simulink model "MorseCode"  (R2013b)
settings: Solver=FixedStepDiscrete  SolverMode=SingleTasking  StartTime=0.0  StopTime=10.0  FixedStep=0.25  RelTol=1e-3
libraries: arduinolib x3
settings Model: ExtModeTrigDuration=2  Creator=ian.alferez  LastModifiedBy=ian.alferez
settings OptimizationCC: OptimizeModelRefInitCode=on  LifeSpan=1
settings DebuggingCC: SolverPrmCheckMsg=none
settings HardwareCC: ProdBitPerInt=16  ProdBitPerPointer=8  ProdIntDivRoundTo=Zero  ProdEndianess=LittleEndian  ProdWordSize=8  ProdHWDeviceType=Atmel->AVR
settings RTWCC: SystemTargetFile=realtime.tlc  GenerateMakefile=off  TemplateMakefile=realtime.tmf  Description=Run on Target Hardware  RTWVerbose=off  ProcessScript=realtime_make_rtw_hook
settings STFCustomTargetCC: TargetLibSuffix=.a  GenerateSampleERTMain=on  ERTCustomFileBanners=on  SupportNonInlinedSFcns=off  SupportVariableSizeSignals=on  MATLABClassNameForMDSCustomization=Simulink.SoftwareTarget.ERTCustomization  GRTInterface=off  SystemTargetFile=realtime.tlc
settings ERTTargetCC: CodeReplacementLibrary=ANSI_C  GenerateSampleERTMain=on  ParMdlRefBuildCompliant=off  CompOptLevelCompliant=off  ConcurrentExecutionCompliant=off  CombineOutputUpdateFcns=off  ERTFirstTimeCompliant=off  SupportContinuousTime=on  SupportVariableSizeSignals=on  ModelStepFunctionPrototypeControlCompliant=off  CPPClassGenCompliant=off  ExtModeTransport=3  ExtModeMexFile=ext_serial_win32_comm  ExtModeMexArgs=0 1 9600  InlinedParameterPlacement=NonHierarchical  ERTSrcFileBannerTemplate=realtime_code_template.cgt  ERTHdrFileBannerTemplate=realtime_code_template.cgt  ERTDataSrcFileTemplate=realtime_code_template.cgt  ERTDataHdrFileTemplate=realtime_code_template.cgt  ERTCustomFileTemplate=realtime_file_process.tlc

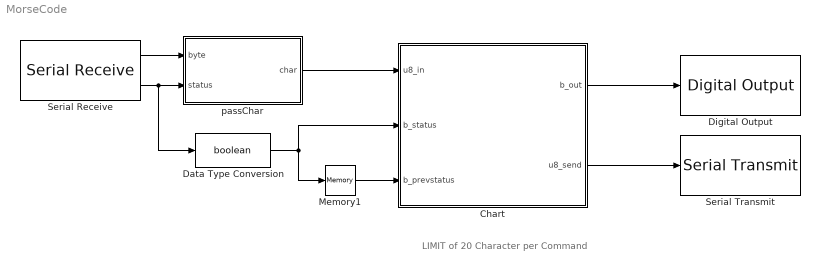
== system MorseCode ==
  note: LIMIT of 20 Character per Command
  Chart : Stateflow chart  TreatAsAtomicUnit=on
  Data Type Conversion : DataTypeConversion  OutDataTypeStr=boolean
  Digital Output : arduinolib/Digital Output  pinNumber=13
  Memory1 : Memory
  Serial Receive : arduinolib/Serial Receive  portNumber=0  showOutStatus=on  sampleTime=0.5
  Serial Transmit : arduinolib/Serial Transmit  portNumber=0
  passChar : MATLAB Function  TreatAsAtomicUnit=on
  wires:
  Serial Receive/2 -> Data Type Conversion/1, passChar/2(status)
  Serial Receive/1 -> passChar/1(byte)
  passChar/1(char) -> Chart/1(u8_in)
  Chart/1(b_out) -> Digital Output/1
  Data Type Conversion/1 -> Memory1/1, Chart/2(b_status)
  Memory1/1 -> Chart/3(b_prevstatus)
  Chart/2(u8_send) -> Serial Transmit/1

== matlab function MorseCode/passChar ==
  data: byte input; char output; status input
function char = passChar(byte,status)
%#codegen
persistent last

if isempty(last)
    last = uint8(0);
end

if (byte>=0 && status == 1)
    last = byte;
else
    byte = last;
end

char = uint8(byte);

== stateflow chart MorseCode/Chart ==
  state SOURCE_MAIN [parallel]
    settings: executionOrder=1
    state RUN
      state STARTUP
      state DONE
        entry:
        b_gotomain = TRUE;
      (default) -> STARTUP : {
          | u8_counter = 0;
          | u8_character[0] = 0;
          | u8_character[1] = 0;
          | u8_character[2] = 0;
          | u8_character[3] = 0;
          | u8_character[4] = 0;
          | u8_character[5] = 0;
          | u8_character[6] = 0;
          | u8_character[7] = 0;
          | u8_character[8] = 0;
          | u8_character[9] = 0;
          | u8_character[10] = 0;
          | u8_character[11] = 0;
          | u8_character[12] = 0;
          | u8_character[13] = 0;
          | u8_character[14] = 0;
          | u8_character[15] = 0;
          | u8_character[16] = 0;
          | u8_character[17] = 0;
          | u8_character[18] = 0;
          | u8_character[19] = 0;
          | }
      STARTUP -> (junction 10)
      (junction 10) -> (junction 3) [order 1] : [b_status == TRUE &&...
          | b_prevstatus == FALSE]
      (junction 10) -> (junction 14) [order 2]
      (junction 3) -> (junction 6) : {
          | u8_character[u8_counter] = u8_in;
          | u8_counter += 1;
          | }
      (junction 6) -> (junction 14) [order 2]
      (junction 6) -> DONE [order 1] : [u8_in == 13]
      (junction 14) -> (junction 39)
    state MAIN
      state Process
        entry:
        b_out = 0;
        u8_count = 0;
        state PULSE
          state IDLE
            b_end = FALSE;
          state SHORT_1
            entry:
            u8_count = 0;
            state OFF
              entry:
              b_out = 0;
            state ON
              entry:
              b_out =1;
              u8_count += 1;
            (default) -> SOURCE_MAIN.MAIN.Process.PULSE.SHORT_1.OFF
            SOURCE_MAIN.MAIN.Process.PULSE.SHORT_1.OFF -> SOURCE_MAIN.MAIN.Process.PULSE.SHORT_1.ON : after(0.25, sec)
            SOURCE_MAIN.MAIN.Process.PULSE.SHORT_1.ON -> SOURCE_MAIN.MAIN.Process.PULSE.SHORT_1.OFF : after(0.25, sec)
          state LONG_1
            entry:
            u8_count = 0;
            state OFF
              entry:
              b_out = 0;
            state ON
              entry:
              b_out =1;
              u8_count += 1;
            (default) -> SOURCE_MAIN.MAIN.Process.PULSE.LONG_1.OFF
            SOURCE_MAIN.MAIN.Process.PULSE.LONG_1.OFF -> SOURCE_MAIN.MAIN.Process.PULSE.LONG_1.ON : after(0.25, sec)
            SOURCE_MAIN.MAIN.Process.PULSE.LONG_1.ON -> SOURCE_MAIN.MAIN.Process.PULSE.LONG_1.OFF : after(1, sec)
          state SHORT_2
            entry:
            u8_count = 0;
            state OFF
              entry:
              b_out = 0;
            state ON
              entry:
              b_out =1;
              u8_count += 1;
            (default) -> SOURCE_MAIN.MAIN.Process.PULSE.SHORT_2.OFF
            SOURCE_MAIN.MAIN.Process.PULSE.SHORT_2.OFF -> SOURCE_MAIN.MAIN.Process.PULSE.SHORT_2.ON : after(0.25, sec)
            SOURCE_MAIN.MAIN.Process.PULSE.SHORT_2.ON -> SOURCE_MAIN.MAIN.Process.PULSE.SHORT_2.OFF : after(0.25, sec)
          state LONG_2
            entry:
            u8_count = 0;
            state OFF
              entry:
              b_out = 0;
            state ON
              entry:
              b_out =1;
              u8_count += 1;
            (default) -> SOURCE_MAIN.MAIN.Process.PULSE.LONG_2.OFF
            SOURCE_MAIN.MAIN.Process.PULSE.LONG_2.OFF -> SOURCE_MAIN.MAIN.Process.PULSE.LONG_2.ON : after(0.25, sec)
            SOURCE_MAIN.MAIN.Process.PULSE.LONG_2.ON -> SOURCE_MAIN.MAIN.Process.PULSE.LONG_2.OFF : after(1, sec)
          state SHORT_3
            entry:
            u8_count = 0;
            state OFF
              entry:
              b_out = 0;
            state ON
              entry:
              b_out =1;
              u8_count += 1;
            (default) -> SOURCE_MAIN.MAIN.Process.PULSE.SHORT_3.OFF
            SOURCE_MAIN.MAIN.Process.PULSE.SHORT_3.OFF -> SOURCE_MAIN.MAIN.Process.PULSE.SHORT_3.ON : after(0.25, sec)
            SOURCE_MAIN.MAIN.Process.PULSE.SHORT_3.ON -> SOURCE_MAIN.MAIN.Process.PULSE.SHORT_3.OFF : after(0.25, sec)
          state LONG_3
            entry:
            u8_count = 0;
            state OFF
              entry:
              b_out = 0;
            state ON
              entry:
              b_out =1;
              u8_count += 1;
            (default) -> SOURCE_MAIN.MAIN.Process.PULSE.LONG_3.OFF
            SOURCE_MAIN.MAIN.Process.PULSE.LONG_3.OFF -> SOURCE_MAIN.MAIN.Process.PULSE.LONG_3.ON : after(0.25, sec)
            SOURCE_MAIN.MAIN.Process.PULSE.LONG_3.ON -> SOURCE_MAIN.MAIN.Process.PULSE.LONG_3.OFF : after(1, sec)
          state SHORT_4
            entry:
            u8_count = 0;
            state OFF
              entry:
              b_out = 0;
            state ON
              entry:
              b_out =1;
              u8_count += 1;
            (default) -> SOURCE_MAIN.MAIN.Process.PULSE.SHORT_4.OFF
            SOURCE_MAIN.MAIN.Process.PULSE.SHORT_4.OFF -> SOURCE_MAIN.MAIN.Process.PULSE.SHORT_4.ON : after(0.25, sec)
            SOURCE_MAIN.MAIN.Process.PULSE.SHORT_4.ON -> SOURCE_MAIN.MAIN.Process.PULSE.SHORT_4.OFF : after(0.25, sec)
          state LONG_4
            entry:
            u8_count = 0;
            state OFF
              entry:
              b_out = 0;
            state ON
              entry:
              b_out =1;
              u8_count += 1;
            (default) -> SOURCE_MAIN.MAIN.Process.PULSE.LONG_4.OFF
            SOURCE_MAIN.MAIN.Process.PULSE.LONG_4.OFF -> SOURCE_MAIN.MAIN.Process.PULSE.LONG_4.ON : after(0.25, sec)
            SOURCE_MAIN.MAIN.Process.PULSE.LONG_4.ON -> SOURCE_MAIN.MAIN.Process.PULSE.LONG_4.OFF : after(1, sec)
          state END
            entry:
            b_end = TRUE;
            u8_count1 += 1;
          (default) -> SOURCE_MAIN.MAIN.Process.PULSE.IDLE
          SOURCE_MAIN.MAIN.Process.PULSE.IDLE -> (junction 48)
          (junction 48) -> (junction 49) [order 1] : [(u8_long1_count > 0) && (u8_short1_count == 0)]
          (junction 48) -> SHORT_1 [order 2]
          (junction 49) -> LONG_1
          SHORT_1 -> (junction 50) : [(u8_count >= u8_short1_count) && (b_out == 0)]
          LONG_1 -> (junction 51) : [(u8_count >= u8_long1_count) && (b_out == 0)]
          (junction 51) -> (junction 50)
          (junction 50) -> (junction 52)
          (junction 52) -> (junction 53) [order 1] : [(u8_long2_count > 0) && (u8_short2_count == 0)]
          (junction 52) -> SHORT_2 [order 2]
          (junction 53) -> LONG_2
          SHORT_2 -> (junction 54) : [(u8_count >= u8_short2_count) && (b_out == 0)]
          LONG_2 -> (junction 55) : [(u8_count >= u8_long2_count) && (b_out == 0)]
          (junction 55) -> (junction 54)
          (junction 54) -> (junction 56)
          (junction 56) -> (junction 57) [order 1] : [(u8_long3_count > 0) && (u8_short3_count == 0)]
          (junction 56) -> SHORT_3 [order 2]
          (junction 57) -> LONG_3
          SHORT_3 -> (junction 58) : [(u8_count >= u8_short3_count) && (b_out == 0)]
          LONG_3 -> (junction 59) : [(u8_count >= u8_long3_count) && (b_out == 0)]
          (junction 59) -> (junction 58)
          (junction 58) -> (junction 60)
          (junction 60) -> (junction 61) [order 1] : [(u8_long4_count > 0) && (u8_short4_count == 0)]
          (junction 60) -> SHORT_4 [order 2]
          (junction 61) -> LONG_4
          SHORT_4 -> (junction 62) : [(u8_count >= u8_short4_count) && (b_out == 0)]
          LONG_4 -> (junction 63) : [(u8_count >= u8_long4_count) && (b_out == 0)]
          (junction 63) -> (junction 62)
          (junction 62) -> END
        (default) -> PULSE : {
            | [u8_long1_count,u8_short1_count,...
            | u8_long2_count,u8_short2_count,...
            | u8_long3_count,u8_short3_count,...
            | u8_long4_count,u8_short4_count] = convert(u8_character[u8_count1]);
            | }
      state IDLE
        entry:
        b_end = FALSE;
      (default) -> SOURCE_MAIN.MAIN.IDLE : {
          | b_end = FALSE;
          | u8_count1 = 0;
          | }
      SOURCE_MAIN.MAIN.IDLE -> Process : [b_end == FALSE]
      Process -> SOURCE_MAIN.MAIN.IDLE : [b_end == TRUE]
    (default) -> RUN : {b_gotomain = FALSE;}
    RUN -> MAIN : [b_gotomain == TRUE]
    MAIN -> (junction 179) : [b_end == TRUE && ...
        | u8_count1 >= u8_counter]
    (junction 179) -> (junction 180) : {
        | b_gotomain = FALSE;
        | }
    (junction 180) -> RUN
  state SOURCE_TRANSMIT [parallel]
    settings: executionOrder=2
    state INIT
    state NEWLINE
      entry:
      u8_send = 10;
    state CHAR
      entry:
      u8_send = u8_in;
    state ENTER
      entry:
      u8_send = 13;
    state NULL
      entry:
      u8_send = 0;
    (default) -> INIT
    INIT -> (junction 215) : [b_status == TRUE &&...
        | b_prevstatus == FALSE]
    (junction 215) -> NEWLINE [order 1] : [u8_in == 13]
    (junction 215) -> CHAR [order 2]
    (junction 231) -> INIT
    NEWLINE -> ENTER
    CHAR -> NULL
    ENTER -> (junction 234)
    NULL -> (junction 231)
    (junction 234) -> NULL
  data: X function_input double; L1 function_output double; S1 function_output double; L2 function_output double; S2 function_output double; L3 function_output double; S3 function_output double; L4 function_output double; S4 function_output double; u8_in input uint8; b_out output uint8 =0; b_status input boolean; TRUE constant boolean =1; b_prevstatus input boolean; FALSE constant boolean =0; u8_counter local uint8; b_end local boolean; u8_character local uint8 size=20; u8_count local uint8; u8_count1 local uint8; u8_long1_count local uint16; u8_long2_count local uint8; u8_long3_count local uint8; u8_long4_count local uint8; u8_short1_count local uint8; u8_short2_count local uint16; u8_short3_count local uint8; u8_short4_count local uint8; b_gotomain local boolean; u8_send output uint8
  function [L1,S1,L2,S2,L3,S3,L4,S4] = convert (X):
    | function [L1,S1,L2,S2,L3,S3,L4,S4] = convert (X)
    | 
    | % initialized the values to zeros
    |     L1 = 0;
    |     S1 = 0;
    |     L2 = 0;
    |     S2 = 0;
    |     L3 = 0;
    |     S3 = 0;
    |     L4 = 0;
    |     S4 = 0;
    |     
    | % in ascii code 97 is"A"
    | X = X - 96;
    | 
    | % A
    | if X == 1
    |     L1 = 0;
    |     S1 = 1;
    |     L2 = 1;
    |     S2 = 0;
    |     L3 = 0;
    |     S3 = 0;
    |     L4 = 0;
    |     S4 = 0;
    | end
    | % B
    | if X == 2
    |     L1 = 1;
    |     S1 = 0;
    |     L2 = 0;
    |     S2 = 3;
    |     L3 = 0;
    |     S3 = 0;
    |     L4 = 0;
    |     S4 = 0;
    | end
    | % C
    | if X == 3
    |     L1 = 1;
    |     S1 = 0;
    |     L2 = 0;
    |     S2 = 1;
    |     L3 = 1;
    |     S3 = 0;
    |     L4 = 0;
    |     S4 = 1;
    | end
    | % D
    | if X == 4
    |     L1 = 1;
    |     S1 = 0;
    |     L2 = 0;
    |     S2 = 2;
    |     L3 = 0;
    |     S3 = 0;
    |     L4 = 0;
    |     S4 = 0;
    | end
    | % E
    | if X == 5
    |     L1 = 0;
    |     S1 = 1;
    |     L2 = 0;
    |     S2 = 0;
    |     L3 = 0;
    |     S3 = 0;
    |     L4 = 0;
    |     S4 = 0;
    | end
    | % F
    | if X == 6
    |     L1 = 0;
    |     S1 = 2;
    |     L2 = 1;
    |     S2 = 0;
    |     L3 = 0;
    |     S3 = 1;
    |     L4 = 0;
    |     S4 = 0;
    | end
    | % G
    | if X == 7
    |     L1 = 2;
    |     S1 = 0;
    |     L2 = 0;
    |     S2 = 1;
    |     L3 = 0;
    |     S3 = 0;
    |     L4 = 0;
    |     S4 = 0;
    | end
    | % H
    | if X == 8
    |     L1 = 0;
    |     S1 = 4;
    |     L2 = 0;
    |     S2 = 0;
    |     L3 = 0;
    |     S3 = 0;
    |     L4 = 0;
    |     S4 = 0;
    | end
    | % I
    | if X == 9
    |     L1 = 0;
    |     S1 = 2;
    |     L2 = 0;
    |     S2 = 0;
    |     L3 = 0;
    |     S3 = 0;
    |     L4 = 0;
    |     S4 = 0;
    | end
    | % J
    | if X == 10
    |     L1 = 0;
    |     S1 = 1;
    |     L2 = 3;
    |     S2 = 0;
    |     L3 = 0;
    |     S3 = 0;
    |     L4 = 0;
    |     S4 = 0;
    | end
    | % K
    | if X == 11
    |     L1 = 1;
    |     S1 = 0;
    |     L2 = 0;
    |     S2 = 1;
    |     L3 = 1;
    |     S3 = 0;
    |     L4 = 0;
    |     S4 = 0;
    | end
    | % L
    | if X == 12
    |     L1 = 0;
    |     S1 = 1;
    |     L2 = 1;
    |     S2 = 2;
    |     L3 = 0;
    |     S3 = 0;
    |     L4 = 0;
    |     S4 = 0;
    | end
    | % M
    | if X == 13
    |     L1 = 2;
    |     S1 = 0;
    |     L2 = 0;
    |     S2 = 0;
    |     L3 = 0;
    |     S3 = 0;
    |     L4 = 0;
    |     S4 = 0;
    | end
    | % N
    | if X == 14
    |     L1 = 1;
    |     S1 = 0;
    |     L2 = 0;
    |     S2 = 1;
    |     L3 = 0;
    |     S3 = 0;
    |     L4 = 0;
    |     S4 = 0;
    | end
    | % O
    | if X == 15
    |     L1 = 3;
    |     S1 = 0;
    |     L2 = 0;
    |     S2 = 0;
    |     L3 = 0;
    |     S3 = 0;
    |     L4 = 0;
    |     S4 = 0;
    | end
    | % P
    | if X == 16
    |     L1 = 0;
    |     S1 = 1;
    |     L2 = 2;
    |     S2 = 0;
    |     L3 = 0;
    |     S3 = 1;
    |     L4 = 0;
    |     S4 = 0;
    | end
    | % Q
    | if X == 17
    |     L1 = 2;
    |     S1 = 0;
    |     L2 = 0;
    |     S2 = 1;
    |     L3 = 1;
    |     S3 = 0;
    |     L4 = 0;
    |     S4 = 0;
    | end
    | % R
    | if X == 18
    |     L1 = 0;
    |     S1 = 1;
    |     L2 = 1;
    |     S2 = 0;
    |     L3 = 0;
    |     S3 = 1;
    |     L4 = 0;
    |     S4 = 0;
    | end
    | % S
    | if X == 19
    |     L1 = 0;
    |     S1 = 3;
    |     L2 = 0;
    |     S2 = 0;
    |     L3 = 0;
    |     S3 = 0;
    |     L4 = 0;
    |     S4 = 0;
    | end
    | % T
    | if X == 20
    |     L1 = 1;
    |     S1 = 0;
    |     L2 = 0;
    |     S2 = 0;
    |     L3 = 0;
    |     S3 = 0;
    |     L4 = 0;
    |     S4 = 0;
    | end
    | % U
    | if X == 21
    |     L1 = 0;
    |     S1 = 2;
    |     L2 = 1;
    |     S2 = 0;
    |     L3 = 0;
    |     S3 = 0;
    |     L4 = 0;
    |     S4 = 0;
    | end
    | % V
    | if X == 22
    |     L1 = 0;
    |     S1 = 3;
    |     L2 = 1;
    |     S2 = 0;
    |     L3 = 0;
    |     S3 = 0;
    |     L4 = 0;
    |     S4 = 0;
    | end
    | % W
    | if X == 23
    |     L1 = 0;
    |     S1 = 1;
    |     L2 = 2;
    |     S2 = 0;
    |     L3 = 0;
    |     S3 = 0;
    |     L4 = 0;
    |     S4 = 0;
    | end
    | % X
    | if X == 24
    |     L1 = 1;
    |     S1 = 0;
    |     L2 = 0;
    |     S2 = 2;
    |     L3 = 1;
    |     S3 = 0;
    |     L4 = 0;
    |     S4 = 0;
    | end
    | % Y
    | if X == 25
    |     L1 = 1;
    |     S1 = 0;
    |     L2 = 0;
    |     S2 = 1;
    |     L3 = 2;
    |     S3 = 0;
    |     L4 = 0;
    |     S4 = 0;
    | end
    | % Z
    | if X == 26
    |     L1 = 2;
    |     S1 = 0;
    |     L2 = 0;
    |     S2 = 2;
    |     L3 = 0;
    |     S3 = 0;
    |     L4 = 0;
    |     S4 = 0;
    | end
    | 
    | 
    | 
    | end
